simulink subsystem "ApplicationOpenLoopSysControl"  (R2024b)
settings: Solver=VariableStepAuto  StartTime=0.0  StopTime=10.0  RelTol=1e-3
settings Model: Creator=The MathWorks, Inc.  LastModifiedBy=The MathWorks, Inc.
settings RTWCC: GPUComputeCapability=3.5

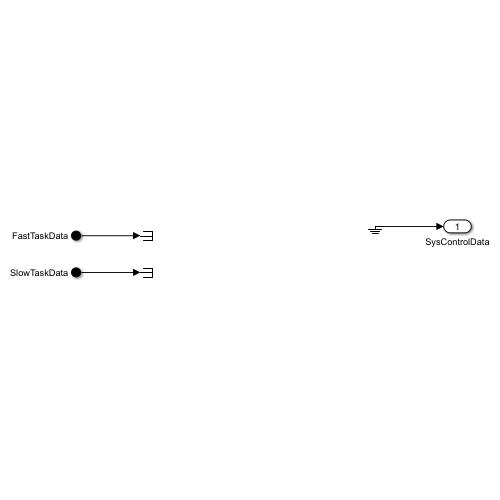
[thumbnail: Simulink's stored preview of the top-level diagram]
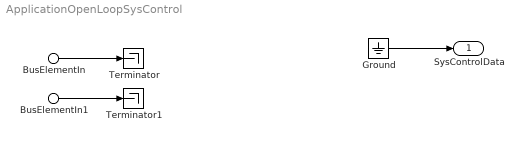
== system ApplicationOpenLoopSysControl ==
  BusElementIn : Inport  PortName=FastTaskData
  BusElementIn1 : Inport  Port=2  PortName=SlowTaskData
  Ground : Ground
  Terminator : Terminator
  Terminator1 : Terminator
  SysControlData : Outport
  wires:
  BusElementIn1/1 -> Terminator1/1
  BusElementIn/1 -> Terminator/1
  Ground/1 -> SysControlData/1
